simulink model "continuous_time_sim"  (R2022a)
settings: Solver=VariableStepAuto  StartTime=0.0  StopTime=5.0  RelTol=1e-3
values from neighbouring files (symbols this model uses):
  A = [0 0 0 0 0 0 40.7055790872 38.6368253303 1 0 -13.2363115295 -4.71950452077 ... (16 elements, 4x4)]    [lin_ss_model.mat]    (also in lin_state_space.m = [0 0     1      0)
  B = [0 0 23.29957643 8.30763585823]    [lin_ss_model.mat]    (also in lin_state_space.m = [0)
  C = eye(2,4)    [LQR_design_realistic.m]    (also in lin_ss_model.mat = [1  0  0  0; 0  1  0  0]; lin_state_space.m; main_LQR_realistic.m = eye(4,4))
  K = 1    [LQR_design_realistic.m]    (also in live_sim.m; main_LQR_realistic.m)
  x0 = [0,0,0,0]    [LQR_design.m]    (also in LQR_design_realistic.m; live_sim.m = x0; main_LQR_realistic.m = [0, disturbance_alpha*pi/180, 0, 0])
  xd = [90*pi/180,0,0,0]    [LQR_design.m]    (also in LQR_design_realistic.m = [30*pi/180,0,0,0]; live_sim.m = xd; main_LQR_realistic.m = xd)
settings Model: Creator=gaetc  LastModifiedBy=gaetc
settings DataIOCC: SaveState=on

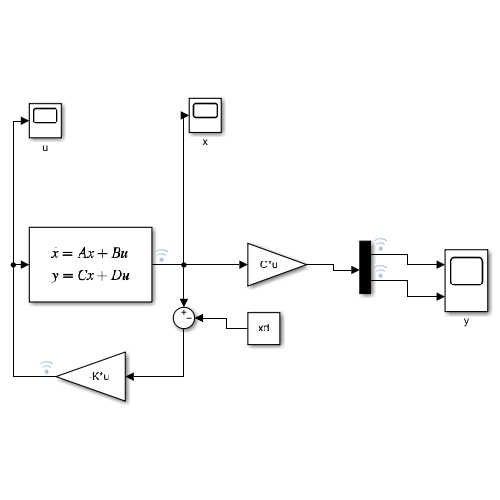
[thumbnail: Simulink's stored preview of the top-level diagram]
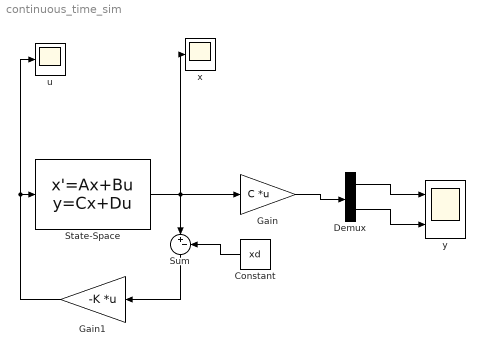
== system continuous_time_sim ==
  Constant : Constant  Value=xd
  Demux : Demux  Outputs=2
  Gain : Gain  Gain=C  Multiplication=Matrix(K*u)
  Gain1 : Gain  Gain=-K  Multiplication=Matrix(K*u)
  State-Space : StateSpace  A=A  B=B  C=eye(4)  D=zeros(4,1)  InitialCondition=x0
  Sum : Sum  Inputs=|+-
  u : Scope
  x : Scope
  y : Scope  NumInputPorts=2
      settings: Tag=theta,alpha
  wires:
  State-Space/1 -> x/1, Gain/1, Sum/1
  Gain1/1 -> u/1, State-Space/1
  Sum/1 -> Gain1/1
  Constant/1 -> Sum/2
  Gain/1 -> Demux/1
  Demux/1 -> y/1
  Demux/2 -> y/2
